simulink model "fwv_modified"  (R2021a)
settings: Solver=ode23t  StartTime=0.0  StopTime=9  FixedStep=0.01  MaxStep=0.01  RelTol=1e-3  AbsTol=1e-3  EnableMultiTasking=on
model workspace: external: MATLAB File param.m (data not in the file)
values from neighbouring files (symbols this model uses):
  A_D = 1.5    [main.m]    (also in param.m; params.m)
  A_L = 1.8    [main.m]    (also in param.m; params.m)
  c_bar = 0.035714285714285712    (= 0.0357142857143)    [main.m]    (also in param.m = 0.0251327412287; params.m)
  C_D0 = 0.45    [main.m]    (also in param.m; params.m)
  f = 37.5    [param.m]
  ht = 4    [main.m]    (also in param.m)
  m = 2    [rbf_pid.m]
  r00 = 0.93333333333333335    (= 0.933333333333)    [main.m]    (also in param.m = 1; params.m)
  r11 = 0.48118518518518516    (= 0.481185185185)    [main.m]    (also in param.m = double(int(curv(x)*(x+1/9),0,1)); params.m)
  r22 = 0.30475061728395064    (= 0.304750617284)    [main.m]    (also in param.m = double(int(curv(x)*(x+1/9)^2,0,1)); params.m)
  r33 = 0.2185686913580247    (= 0.218568691358)    [main.m]    (also in param.m = double(int(curv(x)*(x+1/9)^3,0,1)); params.m)
  r_cp = 0.10758076225045371    (= 0.10758076225)    [main.m]    (also in param.m = Rw*r33/r22; params.m)
  rho = 1.205    [main.m]    (also in param.m; params.m)
  Rw = 0.15    [main.m]    (also in param.m = 0.075; params.m)
  z00 = 1.0017777777777779    (= 1.00177777778)    [main.m]    (also in param.m = double(int(curv(x)^2,0,1)); params.m)
  z11 = 0.48491851851851853    (= 0.484918518519)    [main.m]    (also in param.m = double(int(curv(x)^2*(x+1/9),0,1)); params.m)
  z22 = 0.28785382716049385    (= 0.28785382716)    [main.m]    (also in param.m = double(int(curv(x)^2*(x+1/9)^2,0,1)); params.m)
  zrd = 1.2933386666666666    (= 1.29333866667)    [main.m]    (also in param.m = double(int(curv(x)^4,0,1)); params.m)
undefined symbols (not defined in the file or in its folder): X, Y, Z
libraries: sm_lib x63, nesl_utility x41, vrlib x3, slpidlib x2, simulink x1
(part 3 of 3)

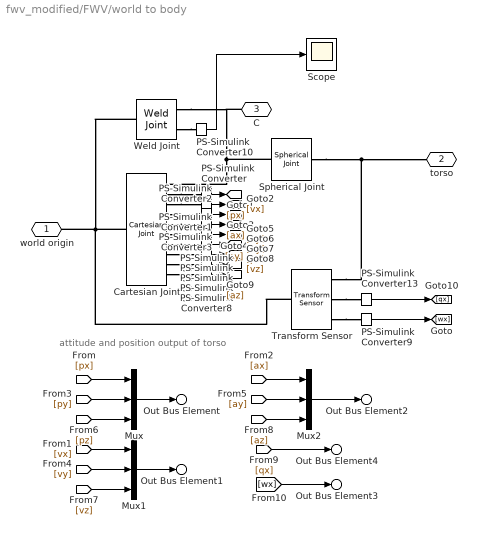
== system fwv_modified/FWV/world to body ==
  note: attitude and position output of torso
  Cartesian Joint : sm_lib/Joints/Cartesian Joint  JointMode=Normal  SenseConstraintForce=off  SenseConstraintForceX=off  SenseConstraintForceY=off  SenseConstraintForceZ=off  SenseConstraintTorque=off  SenseConstraintTorqueX=off  SenseConstraintTorqueY=off  SenseConstraintTorqueZ=off  SenseTotalForce=off  SenseTotalForceX=off  SenseTotalForceY=off  SenseTotalForceZ=off  SenseTotalTorque=off  SenseTotalTorqueX=off  SenseTotalTorqueY=off  SenseTotalTorqueZ=off  CompositeWrenchDir=FollowerOnBase  CompositeWrenchFrame=BaseFrame  PxEquilibriumPosition=0  PxEquilibriumPositionUnits=m  PxSpringStiffness=0  PxSpringStiffnessUnits=N/m  PxDampingCoefficient=0  PxDampingCoefficientUnits=N/(m/s)  PxTorqueActuationMode=NoTorque  PxMotionActuationMode=ComputedMotion  PxSensePosition=on  PxSenseVelocity=on  PxSenseAcceleration=on  PxSenseTorqueForce=off  PxSenseLowerLimitTorqueForce=off  PxSenseUpperLimitTorqueForce=off  PxLowerLimitSpecify=off  PxLowerLimitBound=-1  PxLowerLimitBoundUnits=m  PxLowerLimitStiffness=1e6  PxLowerLimitStiffnessUnits=N/m  PxLowerLimitDamping=1e3  PxLowerLimitDampingUnits=N/(m/s)  PxLowerLimitTransitionRegionWidth=1e-4  PxLowerLimitTransitionRegionWidthUnits=m  PxUpperLimitSpecify=off  PxUpperLimitBound=1  PxUpperLimitBoundUnits=m  PxUpperLimitStiffness=1e6  PxUpperLimitStiffnessUnits=N/m  PxUpperLimitDamping=1e3  PxUpperLimitDampingUnits=N/(m/s)  PxUpperLimitTransitionRegionWidth=1e-4  PxUpperLimitTransitionRegionWidthUnits=m  PxPositionTargetSpecify=off  PxPositionTargetPriority=High  PxPositionTargetValue=0  PxPositionTargetValueUnits=m  PxVelocityTargetSpecify=off  PxVelocityTargetPriority=High  PxVelocityTargetValue=0  PxVelocityTargetValueUnits=m/s  PyEquilibriumPosition=0  PyEquilibriumPositionUnits=m  PySpringStiffness=0  PySpringStiffnessUnits=N/m  PyDampingCoefficient=0  PyDampingCoefficientUnits=N/(m/s)  PyTorqueActuationMode=NoTorque  PyMotionActuationMode=ComputedMotion  PySensePosition=on  PySenseVelocity=on  PySenseAcceleration=on  PySenseTorqueForce=off  PySenseLowerLimitTorqueForce=off  PySenseUpperLimitTorqueForce=off  PyLowerLimitSpecify=off  PyLowerLimitBound=-1  PyLowerLimitBoundUnits=m  PyLowerLimitStiffness=1e6  PyLowerLimitStiffnessUnits=N/m  PyLowerLimitDamping=1e3  PyLowerLimitDampingUnits=N/(m/s)  PyLowerLimitTransitionRegionWidth=1e-4  PyLowerLimitTransitionRegionWidthUnits=m  PyUpperLimitSpecify=off  PyUpperLimitBound=1  PyUpperLimitBoundUnits=m  PyUpperLimitStiffness=1e6  PyUpperLimitStiffnessUnits=N/m  PyUpperLimitDamping=1e3  PyUpperLimitDampingUnits=N/(m/s)  PyUpperLimitTransitionRegionWidth=1e-4  PyUpperLimitTransitionRegionWidthUnits=m  PyPositionTargetSpecify=off  PyPositionTargetPriority=High  PyPositionTargetValue=0  PyPositionTargetValueUnits=m  PyVelocityTargetSpecify=off  PyVelocityTargetPriority=High  PyVelocityTargetValue=0  PyVelocityTargetValueUnits=m/s  PzEquilibriumPosition=0  PzEquilibriumPositionUnits=m  PzSpringStiffness=0  PzSpringStiffnessUnits=N/m  PzDampingCoefficient=0  PzDampingCoefficientUnits=N/(m/s)  PzTorqueActuationMode=NoTorque  PzMotionActuationMode=ComputedMotion  PzSensePosition=on  PzSenseVelocity=on  PzSenseAcceleration=on  PzSenseTorqueForce=off  PzSenseLowerLimitTorqueForce=off  PzSenseUpperLimitTorqueForce=off  PzLowerLimitSpecify=off  PzLowerLimitBound=-1  PzLowerLimitBoundUnits=m  PzLowerLimitStiffness=1e6  PzLowerLimitStiffnessUnits=N/m  PzLowerLimitDamping=1e3  PzLowerLimitDampingUnits=N/(m/s)  PzLowerLimitTransitionRegionWidth=1e-4  PzLowerLimitTransitionRegionWidthUnits=m  PzUpperLimitSpecify=off  PzUpperLimitBound=1  PzUpperLimitBoundUnits=m  PzUpperLimitStiffness=1e6  PzUpperLimitStiffnessUnits=N/m  PzUpperLimitDamping=1e3  PzUpperLimitDampingUnits=N/(m/s)  PzUpperLimitTransitionRegionWidth=1e-4  PzUpperLimitTransitionRegionWidthUnits=m  PzPositionTargetSpecify=on  PzPositionTargetPriority=High  PzPositionTargetValue=z0  PzPositionTargetValueUnits=m  PzVelocityTargetSpecify=off  PzVelocityTargetPriority=High  PzVelocityTargetValue=0  PzVelocityTargetValueUnits=m/s
  Mux : Mux  Inputs=3
  Mux1 : Mux  Inputs=3
  Mux2 : Mux  Inputs=3
  PS-Simulink Converter{,1..10,13} (12 alike) : nesl_utility/PS-Simulink Converter  PhysicalDomain=network_engine_domain  SubClassName=ps_output  LeftPortType=input  RightPortType=output  PseudoPeriodic=off  Frequencies=[]  Unit=inherit  AffineConversion=off
      settings: SourceProductBaseCode=PW,SS
  Scope : Scope
  Spherical Joint : sm_lib/Joints/Spherical Joint  JointMode=Normal  SenseConstraintForce=off  SenseConstraintForceX=off  SenseConstraintForceY=off  SenseConstraintForceZ=off  SenseConstraintTorque=off  SenseConstraintTorqueX=off  SenseConstraintTorqueY=off  SenseConstraintTorqueZ=off  SenseTotalForce=off  SenseTotalForceX=off  SenseTotalForceY=off  SenseTotalForceZ=off  SenseTotalTorque=off  SenseTotalTorqueX=off  SenseTotalTorqueY=off  SenseTotalTorqueZ=off  CompositeWrenchDir=FollowerOnBase  CompositeWrenchFrame=BaseFrame  DefPosRotationMethod=None  DefPosRotationAngleUnits=deg  DefPosRotationStandardAxis=+Z  DefPosRotationAngle=0.0  DefPosRotationArbitraryAxis=[0 0 1]  DefPosFollAlignAxisA=+X  DefPosBaseAlignAxisA=+Y  DefPosFollAlignAxisB=+Y  DefPosBaseAlignAxisB=+Z  DefPosRotationSequenceAxes=FollowerAxes  DefPosRotationSequence=XYX  DefPosRotationSequenceAngles=[0 0 0]  DefPosRotationSequenceAnglesUnits=deg  DefPosRotationMatrix=[1 0 0; 0 1 0; 0 0 1]  EqPosRotationMethod=None  EqPosRotationAngleUnits=deg  EqPosRotationStandardAxis=+Z  EqPosRotationAngle=0.0  EqPosRotationArbitraryAxis=[0 0 1]  EqPosFollAlignAxisA=+X  EqPosBaseAlignAxisA=+Y  EqPosFollAlignAxisB=+Y  EqPosBaseAlignAxisB=+Z  EqPosRotationSequenceAxes=FollowerAxes  EqPosRotationSequence=XYX  EqPosRotationSequenceAngles=[0 0 0]  EqPosRotationSequenceAnglesUnits=deg  EqPosRotationMatrix=[1 0 0; 0 1 0; 0 0 1]  SpringStiffness=0  SpringStiffnessUnits=N*m/deg  DampingCoefficient=0  DampingCoefficientUnits=N*m/(deg/s)  ActuateTorqueX=off  ActuateTorqueY=off  ActuateTorqueZ=off  ActuateTorque=off  TorqueActuationMode=NoTorque  MotionActuationMode=ComputedMotion  ActuationFrame=BaseFrame  SensePosition=off  SenseVelocityX=off  SenseVelocityY=off  SenseVelocityZ=off  SenseVelocity=off  SenseAccelerationX=off  SenseAccelerationY=off  SenseAccelerationZ=off  SenseAcceleration=off  SenseTorqueX=off  SenseTorqueY=off  SenseTorqueZ=off  SenseTorqueForce=off  SenseLowerLimitTorqueMag=off  SenseUpperLimitTorqueMag=off  SensingFrame=BaseFrame  LowerLimitSpecify=off  LowerLimitBound=15  LowerLimitBoundUnits=deg  LowerLimitStiffness=1e4  LowerLimitStiffnessUnits=N*m/deg  LowerLimitDamping=10  LowerLimitDampingUnits=N*m/(deg/s)  LowerLimitTransitionRegionWidth=0.1  LowerLimitTransitionRegionWidthUnits=deg  UpperLimitSpecify=off  UpperLimitBound=45  UpperLimitBoundUnits=deg  UpperLimitStiffness=1e4  UpperLimitStiffnessUnits=N*m/deg  UpperLimitDamping=10  UpperLimitDampingUnits=N*m/(deg/s)  UpperLimitTransitionRegionWidth=0.1  UpperLimitTransitionRegionWidthUnits=deg  PositionTargetRotationMethod=RotationSequence  PositionTargetRotationAngleUnits=deg  PositionTargetRotationStandardAxis=+Z  PositionTargetRotationAngle=0.0  PositionTargetRotationArbitraryAxis=[0 0 1]  PositionTargetFollAlignAxisA=+X  PositionTargetBaseAlignAxisA=+Y  PositionTargetFollAlignAxisB=+Y  PositionTargetBaseAlignAxisB=+Z  PositionTargetRotationSequenceAxes=FollowerAxes  PositionTargetRotationSequence=ZYX  PositionTargetRotationSequenceAngles=[r0 q0 p0]  PositionTargetRotationSequenceAnglesUnits=deg  PositionTargetRotationMatrix=[1 0 0; 0 1 0; 0 0 1]  PositionTargetSpecify=on  PositionTargetPriority=High  VelocityTargetValue=[0 0 0]  VelocityTargetValueUnits=deg/s  VelocityTargetSpecify=off  VelocityTargetPriority=High  VelocityTargetInFollowerFrame=on
  Transform Sensor : sm_lib/Frames and Transforms/Transform Sensor  MeasurementFrame=NonRotatingBase  SenseAngle=off  SenseAxis=off  SenseAngle1=off  SenseAngle2=off  SenseAngle3=off  SenseQ=off  SenseR=on  SenseOmegaX=off  SenseOmegaY=off  SenseOmegaZ=off  SenseOmega1=off  SenseOmega2=off  SenseOmega3=off  SenseQDot=off  SenseRDot=on  SenseAlphaX=off  SenseAlphaY=off  SenseAlphaZ=off  SenseAlpha1=off  SenseAlpha2=off  SenseAlpha3=off  SenseQDDot=off  SenseRDDot=off  SenseX=off  SenseY=off  SenseZ=off  SenseRad=off  SenseAzim=off  SenseDist=off  SenseInc=off  SenseXDot=off  SenseYDot=off  SenseZDot=off  SenseRadDot=off  SenseAzimDot=off  SenseDistDot=off  SenseIncDot=off  SenseXDDot=off  SenseYDDot=off  SenseZDDot=off  SenseRadDDot=off  SenseAzimDDot=off  SenseDistDDot=off  SenseIncDDot=off
  Weld Joint : sm_lib/Joints/Weld Joint  JointMode=Normal  SenseConstraintForce=off  SenseConstraintForceX=off  SenseConstraintForceY=off  SenseConstraintForceZ=off  SenseConstraintTorque=off  SenseConstraintTorqueX=off  SenseConstraintTorqueY=off  SenseConstraintTorqueZ=off  SenseTotalForce=on  SenseTotalForceX=off  SenseTotalForceY=off  SenseTotalForceZ=off  SenseTotalTorque=off  SenseTotalTorqueX=off  SenseTotalTorqueY=off  SenseTotalTorqueZ=off  CompositeWrenchDir=FollowerOnBase  CompositeWrenchFrame=BaseFrame
  world origin : PMIOPort  Side=Left
  torso : PMIOPort  Port=2  Side=Right
  C : PMIOPort  Port=3  Side=Left
  Out Bus Element : Outport  PortName=torso_  Element=p
  Out Bus Element1 : Outport  PortName=torso_  Element=v
  Out Bus Element2 : Outport  PortName=torso_  Element=a
  Out Bus Element3 : Outport  PortName=torso_  Element=Rd
  Out Bus Element4 : Outport  PortName=torso_  Element=R
  wires:
  [vy] -> Mux1/2
  [px] -> Mux/1
  [ax] -> Mux2/1
  [vz] -> Mux1/3
  Mux1/1 -> Out Bus Element1/1
  [az] -> Mux2/3
  [vx] -> Mux1/1
  [ay] -> Mux2/2
  [pz] -> Mux/3
  Mux/1 -> Out Bus Element/1
  Mux2/1 -> Out Bus Element2/1
  [py] -> Mux/2
  PS-Simulink Converter7/1 -> [vz]
  PS-Simulink Converter4/1 -> [vy]
  PS-Simulink Converter5/1 -> [ay]
  PS-Simulink Converter1/1 -> [vx]
  PS-Simulink Converter3/1 -> [py]
  PS-Simulink Converter/1 -> [px]
  PS-Simulink Converter2/1 -> [ax]
  PS-Simulink Converter6/1 -> [pz]
  PS-Simulink Converter8/1 -> [az]
  [qx] -> Out Bus Element4/1
  PS-Simulink Converter13/1 -> [qx]
  PS-Simulink Converter9/1 -> [wx]
  [wx] -> Out Bus Element3/1
  PS-Simulink Converter10/1 -> Scope/1
  connections:
  Transform Sensor/RConn1 -- Spherical Joint/RConn1 -- torso/RConn1
  Spherical Joint/LConn1 -- Weld Joint/RConn1 -- C/RConn1 -- Cartesian Joint/RConn1
  Transform Sensor/RConn2 -- PS-Simulink Converter13/LConn1
  Cartesian Joint/RConn2 -- PS-Simulink Converter/LConn1
  Transform Sensor/RConn3 -- PS-Simulink Converter9/LConn1
  Cartesian Joint/RConn3 -- PS-Simulink Converter1/LConn1
  Cartesian Joint/RConn4 -- PS-Simulink Converter2/LConn1
  Cartesian Joint/RConn5 -- PS-Simulink Converter3/LConn1
  Cartesian Joint/RConn6 -- PS-Simulink Converter4/LConn1
  Cartesian Joint/RConn7 -- PS-Simulink Converter5/LConn1
  Cartesian Joint/RConn8 -- PS-Simulink Converter6/LConn1
  Cartesian Joint/RConn9 -- PS-Simulink Converter7/LConn1
  Cartesian Joint/RConn10 -- PS-Simulink Converter8/LConn1
  Transform Sensor/LConn1 -- world origin/RConn1 -- Weld Joint/LConn1 -- Cartesian Joint/LConn1
  Weld Joint/RConn2 -- PS-Simulink Converter10/LConn1

== system fwv_modified/Controller/Inner PD/get D ==
  In1 : Inport
  Mux : Mux  Inputs=3
  Selector : Selector  NumberOfDimensions=2  InputPortWidth=3  IndexOptions=Index vector (dialog),Index vector (dialog)  Indices=3,2  OutputSizes=1,1
  Selector1 : Selector  NumberOfDimensions=2  InputPortWidth=3  IndexOptions=Index vector (dialog),Index vector (dialog)  Indices=1,3  OutputSizes=1,1
  Selector2 : Selector  NumberOfDimensions=2  InputPortWidth=3  IndexOptions=Index vector (dialog),Index vector (dialog)  Indices=2,1  OutputSizes=1,1
  Transfer Fcn : TransferFcn  Denominator=[1/f 1]
  omega : Outport
  wires:
  In1/1 -> Selector2/1, Selector1/1, Selector/1
  Selector/1 -> Mux/1
  Selector2/1 -> Mux/3
  Mux/1 -> omega/1
  Selector1/1 -> Transfer Fcn/1
  Transfer Fcn/1 -> Mux/2

== system fwv_modified/Controller/Inner PD/get P ==
  eR : Inport
  Add : Sum  Inputs=+++
  Cross Product : vrlib/Utilities/Cross Product
  Cross Product1 : vrlib/Utilities/Cross Product
  Cross Product2 : vrlib/Utilities/Cross Product
  One : Constant  Value=[1;0;0]  OutDataTypeStr=Inherit: Inherit via back propagation
  One1 : Constant  Value=[0;1;0]  OutDataTypeStr=Inherit: Inherit via back propagation
  One2 : Constant  Value=[0;0;1]  OutDataTypeStr=Inherit: Inherit via back propagation
  Product : Product  Multiplication=Matrix(*)
  Product1 : Product  Multiplication=Matrix(*)
  Product2 : Product  Multiplication=Matrix(*)
  Out : Outport
  wires:
  One/1 -> Product/2, Cross Product/1
  One1/1 -> Cross Product1/1, Product1/2
  One2/1 -> Cross Product2/1, Product2/2
  eR/1 -> Product/1, Product1/1, Product2/1
  Cross Product/1 -> Add/1
  Cross Product1/1 -> Add/2
  Cross Product2/1 -> Add/3
  Add/1 -> Out/1
  Product/1 -> Cross Product/2
  Product1/1 -> Cross Product1/2
  Product2/1 -> Cross Product2/2

== system fwv_modified/Controller/Inner PD/to euler1 ==
  R : Inport
  Mux : Mux  Inputs=3
  R to X-Y-Z Extrinsic : Subsystem  mask(Rotation Matrix to X-Y-Z Extrinsic){}
      mask help: Computes roll / pitch / yaw values assuming they correspond to X, Y, and Z rotations, applied in that order and using extrinsic rotations (rotations applied about the fixed axes of the base frame). Does not handle case where Y (pitch) rotation is +/-90 degrees.
  Terminator : Terminator
  rad2deg : Gain  Gain=180/pi
  wires:
  rad2deg/1 -> Terminator/1
  R/1 -> R to X-Y-Z Extrinsic/1(R)
  Mux/1 -> rad2deg/1
  R to X-Y-Z Extrinsic/3(yaw) -> Mux/3
  R to X-Y-Z Extrinsic/1(roll) -> Mux/1
  R to X-Y-Z Extrinsic/2(pitch) -> Mux/2

== system fwv_modified/Controller/Outer PID/x PID1 ==
  In1 : Inport
  In2 : Inport  Port=2
  In3 : Inport  Port=3
  Add : Sum  Inputs=++++
  Constant : Constant  Value=Kp
  Constant1 : Constant  Value=Ki
  Gain : Gain
  Integrator Limited : Integrator  UpperSaturationLimit=1  LowerSaturationLimit=0
  Kd : Step  Time=0  After=Kd  SampleTime=0
  Product : Product
  Product1 : Product
  Product2 : Product
  Transfer Fcn : TransferFcn  Denominator=[1/f 1]
  Out1 : Outport
  wires:
  Add/1 -> Out1/1
  In1/1 -> Product1/2, Product/2
  Product/1 -> Add/1
  Constant/1 -> Product/1
  Product2/1 -> Add/3
  In2/1 -> Transfer Fcn/1
  Kd/1 -> Product2/1
  Integrator Limited/1 -> Add/2
  Product1/1 -> Integrator Limited/1
  Constant1/1 -> Product1/1
  In3/1 -> Gain/1
  Gain/1 -> Add/4
  Transfer Fcn/1 -> Product2/2

== system fwv_modified/Controller/Outer PID/y PID1 ==
  In1 : Inport
  In2 : Inport  Port=2
  In3 : Inport  Port=3
  Add : Sum  Inputs=++++
  Constant : Constant  Value=Kp
  Constant1 : Constant  Value=Ki
  Gain : Gain
  Integrator Limited : Integrator  UpperSaturationLimit=1  LowerSaturationLimit=0
  Kd : Step  Time=0  After=Kd  SampleTime=0
  Product : Product
  Product1 : Product
  Product2 : Product
  Transfer Fcn : TransferFcn  Denominator=[1/f 1]
  Out1 : Outport
  wires:
  Add/1 -> Out1/1
  In1/1 -> Product1/2, Product/2
  Product/1 -> Add/1
  Constant/1 -> Product/1
  Product2/1 -> Add/3
  In2/1 -> Transfer Fcn/1
  Kd/1 -> Product2/1
  Integrator Limited/1 -> Add/2
  Product1/1 -> Integrator Limited/1
  Constant1/1 -> Product1/1
  In3/1 -> Gain/1
  Gain/1 -> Add/4
  Transfer Fcn/1 -> Product2/2

== system fwv_modified/Controller/Outer PID/z PID1 ==
  In1 : Inport
  In2 : Inport  Port=2
  In3 : Inport  Port=3
  Add : Sum  Inputs=++++
  Constant : Constant  Value=Kp
  Constant1 : Constant  Value=Ki
  Integrator Limited : Integrator  LimitOutput=on  UpperSaturationLimit=50  LowerSaturationLimit=-50
  Kd : Step  Time=0  After=Kd  SampleTime=0
  Product : Product
  Product1 : Product
  Product2 : Product
  Transfer Fcn : TransferFcn  Denominator=[1/f 1]
  Out1 : Outport
  wires:
  Add/1 -> Out1/1
  In1/1 -> Product1/2, Product/2
  Product/1 -> Add/1
  Constant/1 -> Product/1
  Product2/1 -> Add/3
  In2/1 -> Transfer Fcn/1
  Kd/1 -> Product2/1
  Integrator Limited/1 -> Add/2
  Product1/1 -> Integrator Limited/1
  Constant1/1 -> Product1/1
  In3/1 -> Add/4
  Transfer Fcn/1 -> Product2/2

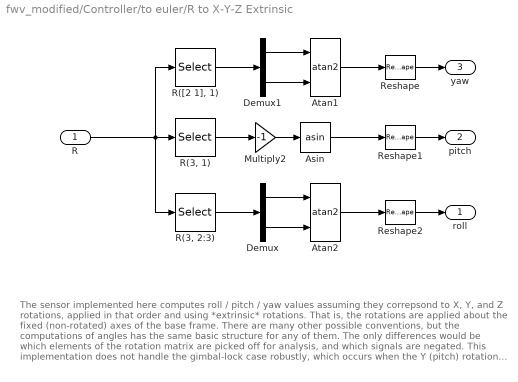
== system fwv_modified/Controller/to euler/R to X-Y-Z Extrinsic ==
  note: The sensor implemented here computes roll / pitch / yaw values assuming they correpsond to X, Y, and Z rotations, applied in that order and using  *extrinsic* rotations.  That is, the rotations are applied about the fixed (non-rotated) axes of the base frame.   There are many other possible conventions, but the computations of angles has the same basic structure for any of them.  The only differences would be which elements of the rotation matrix are picked off for analysis, and which signals are negated.
      |
      | This implementation does not handle the gimbal-lock case robustly, which occurs when the Y (pitch) rotation is +/-90 degrees.  Handling this case requires a more complex computation,
      | but it can be done with a few more trig blocks and selectors.
  R : Inport
  Asin : Trigonometry  Operator=asin
  Atan1 : Trigonometry  Operator=atan2
  Atan2 : Trigonometry  Operator=atan2
  Demux : Demux  Outputs=2
  Demux1 : Demux  Outputs=2
  Multiply2 : Gain  Gain=-1
  "R(3, 1)" : Selector  NumberOfDimensions=2  InputPortWidth=3  IndexOptions=Index vector (dialog),Index vector (dialog)  Indices=3,1  OutputSizes=1,1
  "R(3, 2:3)" : Selector  NumberOfDimensions=2  InputPortWidth=3  IndexOptions=Index vector (dialog),Index vector (dialog)  Indices=3,[2 3]  OutputSizes=1,1
  "R([2 1], 1)" : Selector  NumberOfDimensions=2  InputPortWidth=3  IndexOptions=Index vector (dialog),Index vector (dialog)  Indices=[2 1],1  OutputSizes=1,1
  Reshape : Reshape
  Reshape1 : Reshape
  Reshape2 : Reshape  OutputDimensionality=Customize  OutputDimensions=1
  roll : Outport  VectorParamsAs1DForOutWhenUnconnected=off
  pitch : Outport  Port=2  VectorParamsAs1DForOutWhenUnconnected=off
  yaw : Outport  Port=3  VectorParamsAs1DForOutWhenUnconnected=off
  wires:
  Demux/1 -> Atan2/1
  Demux1/2 -> Atan1/2
  Demux/2 -> Atan2/2
  Atan2/1 -> Reshape2/1
  "R(3, 1)"/1 -> Multiply2/1
  Asin/1 -> Reshape1/1
  R/1 -> "R(3, 1)"/1, "R(3, 2:3)"/1, "R([2 1], 1)"/1
  Demux1/1 -> Atan1/1
  "R([2 1], 1)"/1 -> Demux1/1
  Multiply2/1 -> Asin/1
  "R(3, 2:3)"/1 -> Demux/1
  Atan1/1 -> Reshape/1
  Reshape/1 -> yaw/1
  Reshape1/1 -> pitch/1
  Reshape2/1 -> roll/1

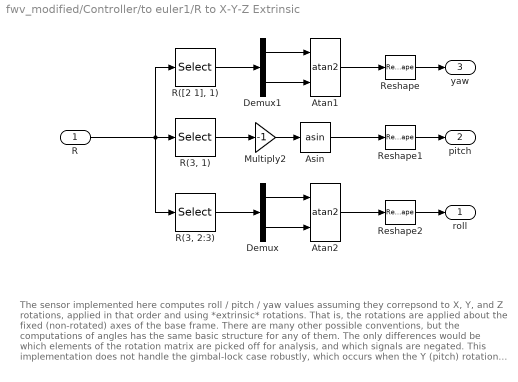
== system fwv_modified/Controller/to euler1/R to X-Y-Z Extrinsic ==
  note: The sensor implemented here computes roll / pitch / yaw values assuming they correpsond to X, Y, and Z rotations, applied in that order and using  *extrinsic* rotations.  That is, the rotations are applied about the fixed (non-rotated) axes of the base frame.   There are many other possible conventions, but the computations of angles has the same basic structure for any of them.  The only differences would be which elements of the rotation matrix are picked off for analysis, and which signals are negated.
      |
      | This implementation does not handle the gimbal-lock case robustly, which occurs when the Y (pitch) rotation is +/-90 degrees.  Handling this case requires a more complex computation,
      | but it can be done with a few more trig blocks and selectors.
  R : Inport
  Asin : Trigonometry  Operator=asin
  Atan1 : Trigonometry  Operator=atan2
  Atan2 : Trigonometry  Operator=atan2
  Demux : Demux  Outputs=2
  Demux1 : Demux  Outputs=2
  Multiply2 : Gain  Gain=-1
  "R(3, 1)" : Selector  NumberOfDimensions=2  InputPortWidth=3  IndexOptions=Index vector (dialog),Index vector (dialog)  Indices=3,1  OutputSizes=1,1
  "R(3, 2:3)" : Selector  NumberOfDimensions=2  InputPortWidth=3  IndexOptions=Index vector (dialog),Index vector (dialog)  Indices=3,[2 3]  OutputSizes=1,1
  "R([2 1], 1)" : Selector  NumberOfDimensions=2  InputPortWidth=3  IndexOptions=Index vector (dialog),Index vector (dialog)  Indices=[2 1],1  OutputSizes=1,1
  Reshape : Reshape
  Reshape1 : Reshape
  Reshape2 : Reshape  OutputDimensionality=Customize  OutputDimensions=1
  roll : Outport  VectorParamsAs1DForOutWhenUnconnected=off
  pitch : Outport  Port=2  VectorParamsAs1DForOutWhenUnconnected=off
  yaw : Outport  Port=3  VectorParamsAs1DForOutWhenUnconnected=off
  wires:
  Demux/1 -> Atan2/1
  Demux1/2 -> Atan1/2
  Demux/2 -> Atan2/2
  Atan2/1 -> Reshape2/1
  "R(3, 1)"/1 -> Multiply2/1
  Asin/1 -> Reshape1/1
  R/1 -> "R(3, 1)"/1, "R(3, 2:3)"/1, "R([2 1], 1)"/1
  Demux1/1 -> Atan1/1
  "R([2 1], 1)"/1 -> Demux1/1
  Multiply2/1 -> Asin/1
  "R(3, 2:3)"/1 -> Demux/1
  Atan1/1 -> Reshape/1
  Reshape/1 -> yaw/1
  Reshape1/1 -> pitch/1
  Reshape2/1 -> roll/1

== system fwv_modified/FWV/LEFT WING/Subsystem1 ==
  Gain : Gain  Gain=-1
  LWing-root in world : sm_lib/Frames and Transforms/Transform Sensor  MeasurementFrame=NonRotatingFollower  SenseAngle=off  SenseAxis=off  SenseAngle1=off  SenseAngle2=off  SenseAngle3=off  SenseQ=off  SenseR=off  SenseOmegaX=on  SenseOmegaY=on  SenseOmegaZ=off  SenseOmega1=off  SenseOmega2=off  SenseOmega3=off  SenseQDot=off  SenseRDot=off  SenseAlphaX=off  SenseAlphaY=off  SenseAlphaZ=off  SenseAlpha1=off  SenseAlpha2=off  SenseAlpha3=off  SenseQDDot=off  SenseRDDot=off  SenseX=off  SenseY=off  SenseZ=off  SenseRad=off  SenseAzim=off  SenseDist=off  SenseInc=off  SenseXDot=on  SenseYDot=on  SenseZDot=off  SenseRadDot=off  SenseAzimDot=off  SenseDistDot=off  SenseIncDot=off  SenseXDDot=off  SenseYDDot=off  SenseZDDot=off  SenseRadDDot=off  SenseAzimDDot=off  SenseDistDDot=off  SenseIncDDot=off
  Mux : Mux
  PS-Simulink Converter{,1..3} (4 alike) : nesl_utility/PS-Simulink Converter  PhysicalDomain=network_engine_domain  SubClassName=ps_output  LeftPortType=input  RightPortType=output  PseudoPeriodic=off  Frequencies=[]  Unit=inherit  AffineConversion=off
      settings: SourceProductBaseCode=PW,SS
  W : PMIOPort  Side=Left
  WT : PMIOPort  Port=2  Side=Left
  le0 : Outport
  wires:
  Mux/1 -> le0/1
  Gain/1 -> Mux/2
  PS-Simulink Converter1/1 -> Mux/3
  PS-Simulink Converter3/1 -> Gain/1
  PS-Simulink Converter2/1 -> Mux/1
  PS-Simulink Converter/1 -> Mux/4
  connections:
  W/RConn1 -- LWing-root in world/LConn1
  WT/RConn1 -- LWing-root in world/RConn1
  LWing-root in world/RConn2 -- PS-Simulink Converter/LConn1
  LWing-root in world/RConn3 -- PS-Simulink Converter1/LConn1
  LWing-root in world/RConn4 -- PS-Simulink Converter2/LConn1
  LWing-root in world/RConn5 -- PS-Simulink Converter3/LConn1

== system fwv_modified/FWV/RIGHT WING/Subsystem1 ==
  Gain : Gain  Gain=-1
  LWing-root in world : sm_lib/Frames and Transforms/Transform Sensor  MeasurementFrame=NonRotatingFollower  SenseAngle=off  SenseAxis=off  SenseAngle1=off  SenseAngle2=off  SenseAngle3=off  SenseQ=off  SenseR=off  SenseOmegaX=on  SenseOmegaY=on  SenseOmegaZ=off  SenseOmega1=off  SenseOmega2=off  SenseOmega3=off  SenseQDot=off  SenseRDot=off  SenseAlphaX=off  SenseAlphaY=off  SenseAlphaZ=off  SenseAlpha1=off  SenseAlpha2=off  SenseAlpha3=off  SenseQDDot=off  SenseRDDot=off  SenseX=off  SenseY=off  SenseZ=off  SenseRad=off  SenseAzim=off  SenseDist=off  SenseInc=off  SenseXDot=on  SenseYDot=on  SenseZDot=off  SenseRadDot=off  SenseAzimDot=off  SenseDistDot=off  SenseIncDot=off  SenseXDDot=off  SenseYDDot=off  SenseZDDot=off  SenseRadDDot=off  SenseAzimDDot=off  SenseDistDDot=off  SenseIncDDot=off
  Mux : Mux
  PS-Simulink Converter{,1..3} (4 alike) : nesl_utility/PS-Simulink Converter  PhysicalDomain=network_engine_domain  SubClassName=ps_output  LeftPortType=input  RightPortType=output  PseudoPeriodic=off  Frequencies=[]  Unit=inherit  AffineConversion=off
      settings: SourceProductBaseCode=PW,SS
  W : PMIOPort  Side=Left
  WT : PMIOPort  Port=2  Side=Left
  le0 : Outport
  wires:
  Mux/1 -> le0/1
  Gain/1 -> Mux/2
  PS-Simulink Converter1/1 -> Mux/3
  PS-Simulink Converter3/1 -> Gain/1
  PS-Simulink Converter2/1 -> Mux/1
  PS-Simulink Converter/1 -> Mux/4
  connections:
  W/RConn1 -- LWing-root in world/LConn1
  WT/RConn1 -- LWing-root in world/RConn1
  LWing-root in world/RConn2 -- PS-Simulink Converter/LConn1
  LWing-root in world/RConn3 -- PS-Simulink Converter1/LConn1
  LWing-root in world/RConn4 -- PS-Simulink Converter2/LConn1
  LWing-root in world/RConn5 -- PS-Simulink Converter3/LConn1

== system fwv_modified/Controller/Inner PD/to euler1/R to X-Y-Z Extrinsic ==
  note: The sensor implemented here computes roll / pitch / yaw values assuming they correpsond to X, Y, and Z rotations, applied in that order and using  *extrinsic* rotations.  That is, the rotations are applied about the fixed (non-rotated) axes of the base frame.   There are many other possible conventions, but the computations of angles has the same basic structure for any of them.  The only differences would be which elements of the rotation matrix are picked off for analysis, and which signals are negated.
      |
      | This implementation does not handle the gimbal-lock case robustly, which occurs when the Y (pitch) rotation is +/-90 degrees.  Handling this case requires a more complex computation,
      | but it can be done with a few more trig blocks and selectors.
  R : Inport
  Asin : Trigonometry  Operator=asin
  Atan1 : Trigonometry  Operator=atan2
  Atan2 : Trigonometry  Operator=atan2
  Demux : Demux  Outputs=2
  Demux1 : Demux  Outputs=2
  Multiply2 : Gain  Gain=-1
  "R(3, 1)" : Selector  NumberOfDimensions=2  InputPortWidth=3  IndexOptions=Index vector (dialog),Index vector (dialog)  Indices=3,1  OutputSizes=1,1
  "R(3, 2:3)" : Selector  NumberOfDimensions=2  InputPortWidth=3  IndexOptions=Index vector (dialog),Index vector (dialog)  Indices=3,[2 3]  OutputSizes=1,1
  "R([2 1], 1)" : Selector  NumberOfDimensions=2  InputPortWidth=3  IndexOptions=Index vector (dialog),Index vector (dialog)  Indices=[2 1],1  OutputSizes=1,1
  Reshape : Reshape
  Reshape1 : Reshape
  Reshape2 : Reshape  OutputDimensionality=Customize  OutputDimensions=1
  roll : Outport  VectorParamsAs1DForOutWhenUnconnected=off
  pitch : Outport  Port=2  VectorParamsAs1DForOutWhenUnconnected=off
  yaw : Outport  Port=3  VectorParamsAs1DForOutWhenUnconnected=off
  wires:
  Demux/1 -> Atan2/1
  Demux1/2 -> Atan1/2
  Demux/2 -> Atan2/2
  Atan2/1 -> Reshape2/1
  "R(3, 1)"/1 -> Multiply2/1
  Asin/1 -> Reshape1/1
  R/1 -> "R(3, 1)"/1, "R(3, 2:3)"/1, "R([2 1], 1)"/1
  Demux1/1 -> Atan1/1
  "R([2 1], 1)"/1 -> Demux1/1
  Multiply2/1 -> Asin/1
  "R(3, 2:3)"/1 -> Demux/1
  Atan1/1 -> Reshape/1
  Reshape/1 -> yaw/1
  Reshape1/1 -> pitch/1
  Reshape2/1 -> roll/1

== matlab function fwv_modified/FWV/RIGHT WING/AoA1 ==
  data: le0 input; alpha output; rot input; Rw parameter; r33 parameter; r22 parameter
function alpha = fcn(le0, rot, Rw, r33, r22)
rcp = -Rw*r33/r22;
vi = le0(1)+le0(3)*rcp;
vo = le0(2)+le0(4)*rcp;
if vi~=0
    alpha = -rot + sign(vi)*pi/2 - atan(vo/vi);
else
    alpha = 0;
end

== matlab function fwv_modified/FWV/RIGHT WING/right aero force and moment ==
  data: le0 input; F_N output; alpha input; M_rd output; d_cp output; rot_dot input; A_L parameter; A_D parameter; C_D0 parameter; rho parameter; c_bar parameter; Rw parameter; r22 parameter; r11 parameter; r00 parameter; z22 parameter; z11 parameter; z00 parameter; zrd parameter
function [F_N,M_rd,d_cp]= fcn(le0, alpha, rot_dot, A_L, A_D, C_D0, rho, c_bar, Rw, r22, r11, r00, z22, z11, z00, zrd)
a2=le0(3)^2+le0(4)^2;
a1=-2*(le0(1)*le0(3)+le0(2)*le0(4));
a0=le0(1)^2+le0(2)^2;
C_L=A_L*sin(2*alpha);
C_D=C_D0+A_D*(1-cos(2*alpha));
C_N=C_L*cos(alpha)+C_D*sin(alpha);
C_A=C_L*sin(alpha)-C_D*cos(alpha);
F_N = -0.5*rho*C_N*c_bar*(a2*Rw^3*r22+a1*Rw^2*r11+a0*Rw*r00);
d_cp_=0.82/pi*(mod(abs(alpha),pi))+0.05;
M_ae=-0.5*rho*C_N*c_bar^2*d_cp_*(a2*Rw^3*z22+a1*Rw^2*z11+a0*Rw*z00);
if F_N==0
    d_cp=-0.51*c_bar;
else
    d_cp=-M_ae/F_N;
end
M_rd=-0.125*rho*5*rot_dot*abs(rot_dot)*Rw*c_bar^4*zrd;

== matlab function fwv_modified/Ref/p,pdot,pddot ==
  data: t input; p output; v output; a output
function [p,v,a] = fcn(t)
% amp=1;
% omega=pi/3;
% hgt=1;
p=[0 0 1];
v=[0 0 0];
a=[0 0 0];
% p(1)=amp*sin(omega*t+pi/2)-amp;
% p(2)=amp*sin(omega*t);
% p(3)=hgt;
% v(1)=amp*omega*sin(omega*t+pi);
% v(2)=amp*omega*sin(omega*t+pi/2);
% v(3)=0;
% a(1)=amp*omega*omega*sin(omega*t+3*pi/2);
% a(2)=amp*omega*omega*sin(omega*t+pi);
% a(3)=0;

== matlab function fwv_modified/Controller/MATLAB Function ==
  data: Rd output; mux input; muy input; muz input; lift output
function [Rd, lift]= fcn(mux, muy, muz)
mu=[mux,muy,9.806];
m=0.02;
lift=m*(muz+9.806);
std_mu=mu./norm(mu);
if norm(std_mu-[0,0,1])<1e-6
    Rd=eye(3);
else
    w=cross([0,0,1],std_mu);
    w=w./norm(w);
    theta=acos(dot([0,0,1],std_mu));
    Rd=axang2rotm([w,theta]);
end

== matlab function fwv_modified/FWV/Signal Input/ left flap ==
  data: t input; y output; amp input; sig input; freq input; bias input
function y = flap(t,amp,sig,freq,bias)
tn = mod(freq*t,1);
if tn<sig
    y = amp*cos(2*pi*tn/(2*sig))+bias;
else
    y = amp*cos(2*pi*(1-tn)/(2-2*sig))+bias;
end
if abs(y)>pi/2
    y = sign(y)*pi/2;
end

== matlab function fwv_modified/FWV/Signal Input/ right flap ==
  data: t input; y output; amp input; sig input; freq input; bias input
function y = flap(t,amp,sig,freq,bias)
sig=1-sig;
tn = mod(freq*t,1);
if tn<sig
    y = amp*cos(2*pi*tn/(2*sig))+bias;
else
    y = amp*cos(2*pi*(1-tn)/(2-2*sig))+bias;
end
if abs(y)>pi/2
    y = sign(y)*pi/2;
end

== matlab function fwv_modified/FWV/LEFT WING/AoA ==
  data: le0 input; alpha output; rot input; Rw parameter; r33 parameter; r22 parameter
function alpha = fcn(le0, rot, Rw, r33, r22)
rcp = Rw*r33/r22;
vi = le0(1)+le0(3)*rcp;
vo = le0(2)+le0(4)*rcp;
dir_v = atan2(vo,vi);
if vi~=0
    alpha = -rot + sign(vi)*pi/2 - atan(vo/vi);
else
    alpha = 0;
end

== matlab function fwv_modified/FWV/LEFT WING/left aero force and moment ==
  data: le0 input; F_N output; alpha input; M_rd output; d_cp output; rot_dot input; A_L parameter; A_D parameter; C_D0 parameter; rho parameter; c_bar parameter; Rw parameter; r22 parameter; r11 parameter; r00 parameter; z22 parameter; z11 parameter; z00 parameter; zrd parameter
function [F_N, M_rd, d_cp] = fcn(le0, alpha, rot_dot, A_L, A_D, C_D0, rho, c_bar, Rw, r22, r11, r00, z22, z11, z00, zrd)
a2=le0(3)^2+le0(4)^2;
a1=2*(le0(1)*le0(3)+le0(2)*le0(4));
a0=le0(1)^2+le0(2)^2;
C_L=A_L*sin(2*alpha);
C_D=C_D0+A_D*(1-cos(2*alpha));
C_N=C_L*cos(alpha)+C_D*sin(alpha);
C_A=C_L*sin(alpha)-C_D*cos(alpha);
F_N = -0.5*rho*C_N*c_bar*(a2*Rw^3*r22+a1*Rw^2*r11+a0*Rw*r00);
d_cp_=0.82/pi*(mod(abs(alpha),pi))+0.05;
M_ae=-0.5*rho*C_N*c_bar^2*d_cp_*(a2*Rw^3*z22+a1*Rw^2*z11+a0*Rw*z00);
if F_N==0
    d_cp=-0.51*c_bar;
else
    d_cp = -M_ae/F_N;
end
M_rd=-0.125*rho*5*rot_dot*abs(rot_dot)*Rw*c_bar^4*zrd;
